simulink model "Ideal_Comparison"  (R2023b)
settings: Solver=VariableStepAuto  StartTime=0.0  StopTime=11  RelTol=1e-3
InitFcn:
  | Ld = 0.000635;
  | Lq = 0.000635;
  | Rs = 0.05;
  | Lambda_m = 0.192;
  | J = 0.011;
  | P = 4;
  | B = 0.001889;
  | Kp = 0.5;
  | Ki = 55;
libraries: slpidlib x6, spsabctodq0Lib x2, SignalEditorBlockLib x1, spspowerguiLib x1
(part 2 of 2)

== system Ideal_Comparison/PMSM2/PMSM Dynamic Model/iqd_calculations ==
  vq : Inport
  Omega_e : Inport  Port=2
  vd : Inport  Port=3
  id_calculations : Subsystem
  iq_calculations : Subsystem
  iq : Outport
  id : Outport  Port=2
  wires:
  vq/1 -> iq_calculations/1(vq)
  id_calculations/1(id) -> id/1, iq_calculations/3(id)
  Omega_e/1 -> iq_calculations/2(Omega_e), id_calculations/2(Omega_e)
  iq_calculations/1(iq) -> iq/1, id_calculations/3(iq)
  vd/1 -> id_calculations/1(vd)

== system Ideal_Comparison/PMSM1/PMSM Dynamic Model/Subsystem/Mechanical_speed_calculations ==
  Te : Inport
  TL : Inport  Port=2
  Add : Sum  Inputs=+--
  Gain : Gain  Gain=(P)*(1/J)
  Gain1 : Gain  Gain=B*(1/P)
  Integrator : Integrator
  Integrator1 : Integrator
  Omega_e : Outport
  Theta_e : Outport  Port=2
  wires:
  Integrator/1 -> Integrator1/1, Omega_e/1, Gain1/1
  Gain/1 -> Integrator/1
  Te/1 -> Add/1
  Add/1 -> Gain/1
  Gain1/1 -> Add/3
  TL/1 -> Add/2
  Integrator1/1 -> Theta_e/1

== system Ideal_Comparison/PMSM1/PMSM Dynamic Model/iqd_calculations/id_calculations ==
  vd : Inport
  Omega_e : Inport  Port=2
  iq : Inport  Port=3
  1/Ld : Gain  Gain=1/Ld
  Add : Sum  Inputs=++-
  Gain : Gain  Gain=Rs
  Integrator : Integrator
  Lq : Gain  Gain=Lq
  Product : Product
  id : Outport
  wires:
  1/Ld/1 -> Integrator/1
  Lq/1 -> Add/2
  vd/1 -> Add/1
  Integrator/1 -> id/1, Gain/1
  Gain/1 -> Add/3
  Add/1 -> 1/Ld/1
  Omega_e/1 -> Product/1
  Product/1 -> Lq/1
  iq/1 -> Product/2

== system Ideal_Comparison/PMSM1/PMSM Dynamic Model/iqd_calculations/iq_calculations ==
  vq : Inport
  Omega_e : Inport  Port=2
  id : Inport  Port=3
  1/Lq : Gain  Gain=1/Lq
  Add : Sum  Inputs=+---
  Gain : Gain  Gain=Rs
  Gain1 : Gain  Gain=Lambda_m
  Integrator : Integrator
  Ld : Gain  Gain=Ld
  Product : Product
  iq : Outport
  wires:
  Integrator/1 -> iq/1, Gain/1
  Add/1 -> 1/Lq/1
  1/Lq/1 -> Integrator/1
  Product/1 -> Ld/1
  vq/1 -> Add/1
  Gain/1 -> Add/4
  Ld/1 -> Add/3
  Omega_e/1 -> Gain1/1, Product/1
  id/1 -> Product/2
  Gain1/1 -> Add/2

== system Ideal_Comparison/PMSM2/PMSM Dynamic Model/Subsystem/Mechanical_speed_calculations ==
  Te : Inport
  TL : Inport  Port=2
  Add : Sum  Inputs=+--
  Gain : Gain  Gain=(P)*(1/J)
  Gain1 : Gain  Gain=B*(1/P)
  Integrator : Integrator
  Integrator1 : Integrator
  Omega_e : Outport
  Theta_e : Outport  Port=2
  wires:
  Integrator/1 -> Integrator1/1, Omega_e/1, Gain1/1
  Gain/1 -> Integrator/1
  Te/1 -> Add/1
  Add/1 -> Gain/1
  Gain1/1 -> Add/3
  TL/1 -> Add/2
  Integrator1/1 -> Theta_e/1

== system Ideal_Comparison/PMSM2/PMSM Dynamic Model/iqd_calculations/id_calculations ==
  vd : Inport
  Omega_e : Inport  Port=2
  iq : Inport  Port=3
  1/Ld : Gain  Gain=1/Ld
  Add : Sum  Inputs=++-
  Gain : Gain  Gain=Rs
  Integrator : Integrator
  Lq : Gain  Gain=Lq
  Product : Product
  id : Outport
  wires:
  1/Ld/1 -> Integrator/1
  Lq/1 -> Add/2
  vd/1 -> Add/1
  Integrator/1 -> id/1, Gain/1
  Gain/1 -> Add/3
  Add/1 -> 1/Ld/1
  Omega_e/1 -> Product/1
  Product/1 -> Lq/1
  iq/1 -> Product/2

== system Ideal_Comparison/PMSM2/PMSM Dynamic Model/iqd_calculations/iq_calculations ==
  vq : Inport
  Omega_e : Inport  Port=2
  id : Inport  Port=3
  1/Lq : Gain  Gain=1/Lq
  Add : Sum  Inputs=+---
  Gain : Gain  Gain=Rs
  Gain1 : Gain  Gain=Lambda_m
  Integrator : Integrator
  Ld : Gain  Gain=Ld
  Product : Product
  iq : Outport
  wires:
  Integrator/1 -> iq/1, Gain/1
  Add/1 -> 1/Lq/1
  1/Lq/1 -> Integrator/1
  Product/1 -> Ld/1
  vq/1 -> Add/1
  Gain/1 -> Add/4
  Ld/1 -> Add/3
  Omega_e/1 -> Gain1/1, Product/1
  id/1 -> Product/2
  Gain1/1 -> Add/2
